simulink model "matrix_loop_stable"  (Simulink 8.1)
settings: Solver=ode45  StartTime=0.0  StopTime=10.0  RelTol=1e-3
settings Model: Creator=dejanira  LastModifiedBy=dejanira
settings DataIOCC: SignalLoggingSaveFormat=Dataset
settings OptimizationCC: ExpressionDepthLimit=128
settings DebuggingCC: FcnCallInpInsideContextMsg=EnableAllAsError
settings GRTTargetCC: CombineOutputUpdateFcns=on  GRTInterface=off

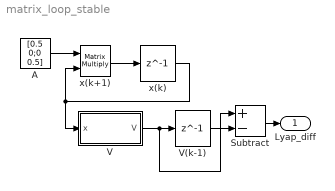
== system matrix_loop_stable ==
  A : Constant  Value=[0.5 0;0 0.5]  VectorParams1D=off
  Subtract : Sum  Inputs=+-
  V : Subsystem
      mask Display: disp('x1^2+x2^2')
  V(k-1) : Delay  DelayLength=1  InitialCondition=100000  SampleTime=0.01
  x(k) : Delay  DelayLength=1
  x(k+1) : Product  Multiplication=Matrix(*)
  Lyap_diff : Outport
  wires:
  A/1 -> x(k+1)/1
  x(k+1)/1 -> x(k)/1
  x(k)/1 -> V/1(x), x(k+1)/2
  V/1(V) -> Subtract/1, V(k-1)/1
  V(k-1)/1 -> Subtract/2
  Subtract/1 -> Lyap_diff/1

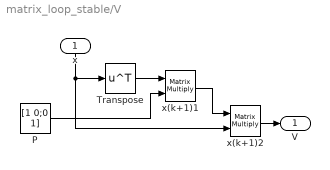
== system matrix_loop_stable/V ==
  x : Inport
  P : Constant  Value=[1 0;0 1]
  Transpose : Math  Operator=transpose  SaturateOnIntegerOverflow=on
  x(k+1)1 : Product  Multiplication=Matrix(*)
  x(k+1)2 : Product  Multiplication=Matrix(*)
  V : Outport
  wires:
  Transpose/1 -> x(k+1)1/1
  x(k+1)1/1 -> x(k+1)2/1
  x/1 -> x(k+1)2/2, Transpose/1
  x(k+1)2/1 -> V/1
  P/1 -> x(k+1)1/2
